simulink model "w2_hw_6DOF"  (R2023b)
settings: Solver=ode45  StartTime=0.0  StopTime=10  MaxStep=0.02  RelTol=1e-5  AbsTol=1e-7
undefined symbols (not defined in the file or in its folder): deg, rad, s
libraries: simulink x6, aerolibconvert2 x4, shared6dof x1
settings Model: Creator=The MathWorks, Inc.  LastModifiedBy=1234
settings SolverCC: AutoScaleAbsTol=off  AlgebraicLoopSolver=TrustRegion
settings DataIOCC: SaveFormat=Array  SaveOutput=off  ReturnWorkspaceOutputs=off
settings OptimizationCC: DefaultParameterBehavior=Inlined  InlineInvariantSignals=on  ReuseModelBlockBuffer=off  ExpressionDepthLimit=2147483647  InitFltsAndDblsToZero=on  EfficientFloat2IntCast=on  LifeSpan=inf
settings DebuggingCC: SaveWithParameterizedLinksMsg=none  MultiTaskCondExecSysMsg=none  SigSpecEnsureSampleTimeMsg=none  FcnCallInpInsideContextMsg=warning  UnconnectedInputMsg=warning  UnconnectedOutputMsg=warning  UnconnectedLineMsg=warning  UniqueDataStoreMsg=error  StateNameClashWarn=warning  StrictBusMsg=ErrorOnBusTreatedAsVector  SFUnexpectedBacktrackingDiag=warning  SFNoUnconditionalDefaultTransitionDiag=warning  SFExecutionAtInitializationDiag=none  ArithmeticOperatorsInVariantConditions=warning
settings HardwareCC: ProdBitPerPointer=32  ProdLargestAtomicFloat=None  ProdIntDivRoundTo=Undefined  ProdEndianess=Unspecified  ProdWordSize=32  ProdHWDeviceType=32-bit Generic  TargetUnknown=on
settings ModelReferenceCC: EnableRefExpFcnMdlSchedulingChecks=on  PropagateSignalLabelsOutOfModel=off
settings SFSimCC: SimUseLocalCustomCode=off  CustomCodeUndefinedFunction=UseInterfaceOnly
settings RTWCC: TemplateMakefile=grt_vc.tmf  RTWUseLocalCustomCode=off
settings CodeAppCC: StateflowObjectComments=on
settings GRTTargetCC: TargetFcnLib=ansi_tfl_tmw.mat  TargetLangStandard=C89/C90 (ANSI)  CombineOutputUpdateFcns=off  GRTInterface=on
settings ConfigComp: CovMetricSettings=d  CovSaveCumulativeToWorkspaceVar=on  CovSaveSingleToWorkspaceVar=on  CovExternalEMLEnable=off

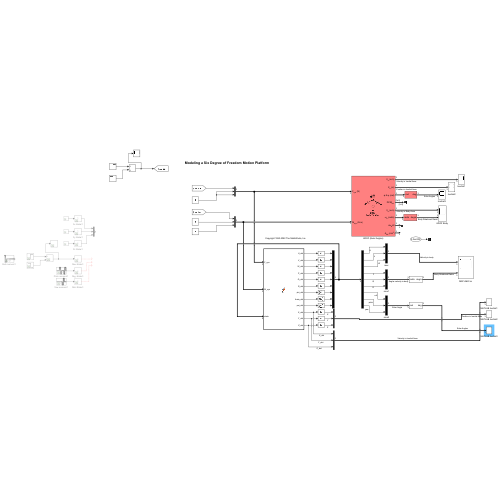
[thumbnail: Simulink's stored preview of the top-level diagram]
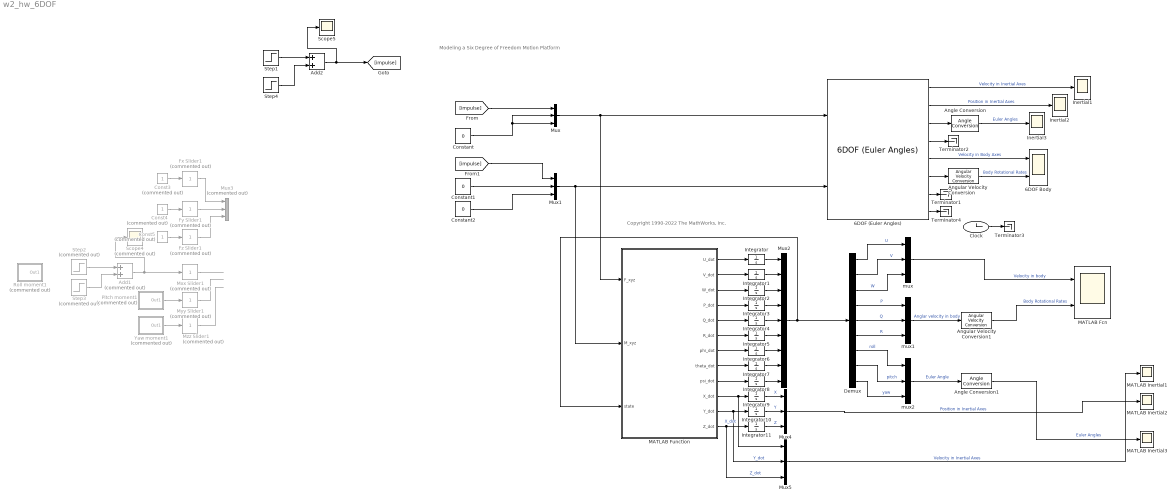
== system w2_hw_6DOF ==
  note: Modeling a Six Degree of Freedom Motion Platform
  note: Copyright 1990-2022 The MathWorks, Inc.
  6DOF (Euler Angles) : shared6dof/6DOF (Euler Angles)  units=Metric (MKS)  mtype=Fixed  rep=Euler Angles  xme_0=[0 0 0]  Vm_0=[0 0 0]  eul_0=[0 0 0]  pm_0=[0 0 0]  mass_0=1.0  mass_e=0.5  mass_f=2.0  inertia=eye(3)  inertia_e=eye(3)  inertia_f=2*eye(3)  k_quat=1.0  vre_flag=on  abi_flag=off  aMode=0  xme_statename=''  Vm_statename=''  eul_statename=''  quat_statename=''  pm_statename=''  mass_statename=''
  6DOF Body : Scope  NumInputPorts=2
  Add1 : Sum  Commented=on
  Add2 : Sum
  Angle Conversion : aerolibconvert2/Angle Conversion  IU=rad  OU=deg
  Angle Conversion1 : aerolibconvert2/Angle Conversion  IU=rad  OU=deg
  Angular Velocity Conversion : aerolibconvert2/Angular Velocity Conversion  IU=rad/s  OU=deg/s
  Angular Velocity Conversion1 : aerolibconvert2/Angular Velocity Conversion  IU=rad/s  OU=deg/s
  Clock : Clock
      settings: Decimation=100
  Const3 : Constant  Commented=on
  Const4 : Constant  Commented=on
  Const5 : Constant  Commented=on
  Constant : Constant  Value=0
  Constant1 : Constant  Value=0
  Constant2 : Constant  Value=0
  Demux : Demux  Outputs=9
  Fx Slider1 : simulink/Math Operations/Slider Gain  Commented=on  gain=1  low=-1  high=1
  Fy Slider1 : simulink/Math Operations/Slider Gain  Commented=on  gain=1  low=-1  high=1
  Fz Slider1 : simulink/Math Operations/Slider Gain  Commented=on  gain=1  low=-1  high=1
  Inertial1 : Scope
  Inertial2 : Scope
  Inertial3 : Scope
  Integrator{,1..5,9..11} (9 alike) : Integrator
  Integrator6 : Integrator  WrapState=on
  Integrator7 : Integrator  WrapState=on
  Integrator8 : Integrator  WrapState=on
  MATLAB Fcn : Scope  NumInputPorts=2
  MATLAB Function : MATLAB Function  TreatAsAtomicUnit=on
  MATLAB Inertial1 : Scope
  MATLAB Inertial2 : Scope
  MATLAB Inertial3 : Scope
  Mux{,1,4..5} (4 alike) : Mux  Inputs=3
  Mux2 : Mux  Inputs=9
  Mux3 : Mux  Commented=on  Inputs=3
  Mxx Slider1 : simulink/Math Operations/Slider Gain  Commented=on  gain=1  low=-5  high=10
  Myy Slider1 : simulink/Math Operations/Slider Gain  Commented=on  gain=1  low=-10  high=10
  Mzz Slider1 : simulink/Math Operations/Slider Gain  Commented=on  gain=1  low=-1  high=1
  Pitch moment1 : Subsystem  Commented=on  mask(timed input){t=[0 3 3 4 4 5 5  7.5 7.5 8.5 8.5 9.5 9.5 10], u=[0 0  1 1 -1 -1.005 0 0 -1 -1 1 1 0 0]*3.138/2}
      mask prompts: t "time values:"; u "input values"
      mask Display: plot(t,u)
  Roll moment1 : Subsystem  Commented=on  mask(timed input){t=[0 1 1 2 2  10], u=[1 1 -1 -.998  0 0]*3.144/2}
      mask prompts: t "time values:"; u "input values"
      mask Display: plot(t,u)
  Scope4 : Scope  Commented=on
  Scope5 : Scope
  Step1 : Step  SampleTime=0
  Step2 : Step  Commented=on  SampleTime=0
  Step3 : Step  Commented=on  Time=1.5  After=-1  SampleTime=0
  Step4 : Step  Time=1.5  After=-1  SampleTime=0
  Terminator{1..4} (4 alike) : Terminator
  Yaw moment1 : Subsystem  Commented=on  mask(timed input){t=[0 6 6 7 7 8 8 10], u=[0 0  -1 -1 1 1 0 0]*3.1/2}
      mask prompts: t "time values:"; u "input values"
      mask Display: plot(t,u)
  mux : Mux  Inputs=3
  mux1 : Mux  Inputs=3
  mux2 : Mux  Inputs=3
  wires:
  Clock/1 -> Terminator3/1
  Mux1/1 -> MATLAB Function/2(M_xyz), 6DOF (Euler Angles)/2
  Mux/1 -> MATLAB Function/1(F_xyz), 6DOF (Euler Angles)/1
  6DOF (Euler Angles)/4 -> Terminator2/1
  6DOF (Euler Angles)/7 -> Terminator1/1
  6DOF (Euler Angles)/3 -> Angle Conversion/1
  6DOF (Euler Angles)/5 -> 6DOF Body/1  "Velocity in Body Axes"
  6DOF (Euler Angles)/1 -> Inertial1/1  "Velocity in Inertial Axes"
  6DOF (Euler Angles)/2 -> Inertial2/1  "Position in Inertial Axes"
  Angle Conversion/1 -> Inertial3/1  "Euler Angles"
  6DOF (Euler Angles)/6 -> Angular Velocity Conversion/1
  Angular Velocity Conversion/1 -> 6DOF Body/2  "Body Rotational Rates"
  6DOF (Euler Angles)/8 -> Terminator4/1
  MATLAB Function/1(U_dot) -> Integrator/1
  MATLAB Function/2(V_dot) -> Integrator1/1
  MATLAB Function/3(W_dot) -> Integrator2/1
  MATLAB Function/4(P_dot) -> Integrator3/1
  MATLAB Function/5(Q_dot) -> Integrator4/1
  MATLAB Function/6(R_dot) -> Integrator5/1
  MATLAB Function/7(phi_dot) -> Integrator6/1
  MATLAB Function/8(theta_dot) -> Integrator7/1
  MATLAB Function/9(psi_dot) -> Integrator8/1
  Integrator/1 -> Mux2/1
  Integrator1/1 -> Mux2/2
  Integrator2/1 -> Mux2/3
  Integrator3/1 -> Mux2/4
  Integrator4/1 -> Mux2/5
  Integrator5/1 -> Mux2/6
  Integrator6/1 -> Mux2/7
  Integrator7/1 -> Mux2/8
  Integrator8/1 -> Mux2/9
  Mux2/1 -> Demux/1, MATLAB Function/3(state)
  Demux/1 -> mux/1  "U"
  Demux/2 -> mux/2  "V"
  Demux/3 -> mux/3  "W"
  mux/1 -> MATLAB Fcn/1  "Velocity in body"
  Demux/4 -> mux1/1  "P"
  Demux/5 -> mux1/2  "Q"
  Demux/6 -> mux1/3  "R"
  mux1/1 -> Angular Velocity Conversion1/1  "Anglar velocity in body"
  Demux/7 -> mux2/1  "roll"
  Demux/8 -> mux2/2  "pitch"
  Demux/9 -> mux2/3  "yaw"
  mux2/1 -> Angle Conversion1/1  "Euler Angle"
  Angular Velocity Conversion1/1 -> MATLAB Fcn/2  "Body Rotational Rates"
  Add1/1 -> Scope4/1, Mxx Slider1/1
  Const5/1 -> Fz Slider1/1
  Mxx Slider1/1 -> ?
  Step3/1 -> Add1/2
  Fz Slider1/1 -> Mux3/3
  Fy Slider1/1 -> Mux3/2
  Mzz Slider1/1 -> ?
  Myy Slider1/1 -> ?
  Fx Slider1/1 -> Mux3/1
  Pitch moment1/1(Out1) -> Myy Slider1/1
  Step2/1 -> Add1/1
  Const4/1 -> Fy Slider1/1
  Const3/1 -> Fx Slider1/1
  Yaw moment1/1(Out1) -> Mzz Slider1/1
  Step4/1 -> Add2/2
  Add2/1 -> Scope5/1, [impulse]
  Step1/1 -> Add2/1
  Constant/1 -> Mux/3, Mux/2
  Constant1/1 -> Mux1/2
  Constant2/1 -> Mux1/3
  [impulse] -> Mux/1
  [impulse] -> Mux1/1
  MATLAB Function/10(X_dot) -> Mux5/1, Integrator9/1  "X_dot"
  MATLAB Function/11(Y_dot) -> Mux5/2, Integrator10/1  "Y_dot"
  MATLAB Function/12(Z_dot) -> Mux5/3, Integrator11/1  "Z_dot"
  Integrator10/1 -> Mux4/2  "Y"
  Integrator9/1 -> Mux4/1  "X"
  Integrator11/1 -> Mux4/3  "Z"
  Mux5/1 -> MATLAB Inertial1/1  "Velocity in Inertial Axes"
  Mux4/1 -> MATLAB Inertial2/1  "Position in Inertial Axes"
  Angle Conversion1/1 -> MATLAB Inertial3/1  "Euler Angles"

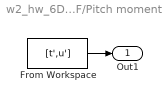
== system w2_hw_6DOF/Pitch moment1 ==
  From Workspace : FromWorkspace  VariableName=[t',u']  ZeroCross=off
  Out1 : Outport  VectorParamsAs1DForOutWhenUnconnected=off
  wires:
  From Workspace/1 -> Out1/1

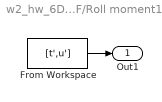
== system w2_hw_6DOF/Roll moment1 ==
  From Workspace : FromWorkspace  VariableName=[t',u']  ZeroCross=off
  Out1 : Outport  VectorParamsAs1DForOutWhenUnconnected=off
  wires:
  From Workspace/1 -> Out1/1

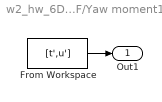
== system w2_hw_6DOF/Yaw moment1 ==
  From Workspace : FromWorkspace  VariableName=[t',u']  ZeroCross=off
  Out1 : Outport  VectorParamsAs1DForOutWhenUnconnected=off
  wires:
  From Workspace/1 -> Out1/1

== matlab function w2_hw_6DOF/MATLAB Function ==
  data: F_xyz input; U_dot output; M_xyz input; state input; V_dot output; W_dot output; P_dot output; Q_dot output; R_dot output; phi_dot output; theta_dot output; psi_dot output; X_dot output; Y_dot output; Z_dot output
function [U_dot, V_dot, W_dot, P_dot, Q_dot, R_dot, phi_dot, theta_dot, psi_dot, X_dot, Y_dot, Z_dot] = fcn(F_xyz, M_xyz, state)

%% Constants
m = 1; % mass
I = [1 0 0;
     0 1 1;
     0 0 1]; %MOI



%% Code - DO NOT EDIT

Ixx = I(1,1); Ixy = I(1,2); Ixz = I(1,3);
Iyx = I(2,1); Iyy = I(2,2); Iyz = I(2,3);
Izx = I(3,1); Izy = I(3,2); Izz = I(3,3);

Fx = F_xyz(1);
Fy = F_xyz(2);
Fz = F_xyz(3);
    
L = M_xyz(1);
M = M_xyz(2);   
N = M_xyz(3);

U = state(1); %[m/s]
V = state(2); %[m/s]
W = state(3); %[m/s]
P = state(4); % [rad/s]
Q = state(5); % [rad/s]
R = state(6); % [rad/s] 
phi = state(7); % pi [rad]
theta = state(8); % theta [rad]
psi = state(9); % psi [rad]


%% OUTPUT
%U_dot = V*R - W*Q - g*sin(pitch) + 1/m*Fx;
%V_dot = W*P - U*R + g*sin(roll)*cos(pitch) + 1/m*Fy;
%W_dot = U*Q - W*P + g*cos(roll)*cos(pitch) + 1/m*Fz; with gravity

U_dot = V*R - W*Q  + 1/m*Fx;
V_dot = W*P - U*R  + 1/m*Fy;
W_dot = U*Q - V*P  + 1/m*Fz;

gam = Izz-Ixz^2/Ixx;
R_dot = N/gam + Ixz/Ixx*1/gam*L - 1/gam*(Iyy-Ixx-Ixz^2/Ixx)*P*Q - Ixz/gam*(1-(Iyy-Izz)/Ixx)*Q*R;
P_dot = L/Ixx + Ixz*R_dot + Ixz/Ixx*P*Q + (Iyy-Izz)/Ixx*Q*R;
Q_dot = M/Iyy - (Ixx-Izz)/Iyy*P*R - Ixz/Iyy*(P^2-R^2);
phi_dot = P + Q*sin(phi)*sin(theta) + R*cos(phi)*tan(theta);
theta_dot = Q*cos(phi) - R*sin(phi);
psi_dot = Q*sin(phi)*sec(theta) + R*cos(phi)*sec(theta);


X_dot = (cos(theta)*cos(psi))*U + (sin(phi)*sin(theta)*cos(psi) - cos(phi)*sin(psi))*V + (cos(phi)*sin(theta)*cos(psi) + sin(phi)*sin(psi))*W;
Y_dot = (cos(theta)*sin(psi))*U + (sin(phi)*sin(theta)*sin(psi) + cos(phi)*cos(psi))*V + (cos(phi)*sin(theta)*sin(psi)-sin(phi)*cos(psi))*W;
Z_dot = -(sin(theta))*U + (sin(phi)*cos(theta))*V + (cos(phi)*cos(theta))*W;
